simulink model "IndicatingResistor_Test"  (R2019a)
settings: Solver=VariableStepAuto  StartTime=0.0  StopTime=10.0  RelTol=1e-3
libraries: Murphy_SimscapeElectrical x6, fl_lib x1, nesl_utility x1, ee_lib x1
settings Model: Creator=Matt  LastModifiedBy=Matt
settings SimscapeCC: SimscapeLogType=all

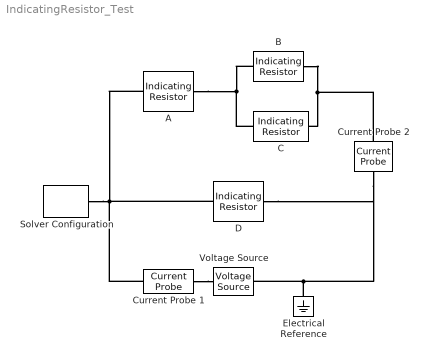
== system IndicatingResistor_Test ==
  A : Murphy_SimscapeElectrical/Indicating Resistor  amps=0.6  volts=6  resistance=10
      settings: SourceProductName=Simscape Electrical - Murphy Utilities
  B : Murphy_SimscapeElectrical/Indicating Resistor  amps=0.3  volts=3  resistance=10
      settings: SourceProductName=Simscape Electrical - Murphy Utilities
  C : Murphy_SimscapeElectrical/Indicating Resistor  amps=0.3  volts=3  resistance=10
      settings: SourceProductName=Simscape Electrical - Murphy Utilities
  Current Probe 1 : Murphy_SimscapeElectrical/Current Probe 
      settings: SourceProductName=Simscape Electrical - Murphy Utilities
  Current Probe 2 : Murphy_SimscapeElectrical/Current Probe 
      settings: SourceProductName=Simscape Electrical - Murphy Utilities
  D : Murphy_SimscapeElectrical/Indicating Resistor  amps=0.9  volts=9  resistance=10
      settings: SourceProductName=Simscape Electrical - Murphy Utilities
  Electrical Reference : fl_lib/Electrical/Electrical Elements/Electrical Reference
  Solver Configuration : nesl_utility/Solver Configuration  PhysicalDomain=network_engine_domain  SubClassName=solver  LeftPortType=input  RightPortType=generic  Tones=[]  Harmonics=[]  SimulateNoise=off  Profile=off  UseLocalSampling=off  EnableSwitchedLinearOptims=on  FrequencyDomain=off  UseCCode=off  RelTol=0.001  AbsTol=1e-06  MinStep=1e-09  ToWorkspace=off  RevertToSquareIcSolve=off  NumHomotopyIterations=100  PhasorMode=off  PhasorModeNumHarmonics=1  DoDC=on  ResidualTolerance=1e-09  UseLocalSolver=off  LocalSolverChoice=NE_BACKWARD_EULER_ADVANCER  LocalSolverSampleTime=0.001  DoFixedCost=off  MaxNonlinIter=3  MaxModeIter=2  LinearAlgebra=auto  EquationFormulation=NE_TIME_EF  DelaysMemoryBudget=1024  AutomaticFiltering=on  FilteringTimeConstant=0.001  PartitionStorageMethod=AS_NEEDED  PartitionMemoryBudget=1024  PartitionMethod=ROBUST
  Voltage Source : ee_lib/Sources/Voltage Source  dc_voltage=9 V  ac_voltage=0 V  ac_shift=0 rad  ac_frequency=60 Hz  noise_mode=0  PSD=0 V^2/Hz  repeatability=1  auto_seed=3394773151  user_seed=0  sample_time=1e-3 s  i_specify=off  i_priority=None  i=0 A  i_nominal_specify=off  i_nominal_unit=A  i_nominal_value=1  v_specify=off  v_priority=None  v=0 V  v_nominal_specify=off  v_nominal_unit=V  v_nominal_value=1
      settings: SourceProductName=Simscape Electrical
  connections:
  Electrical Reference/LConn1 -- D/RConn1 -- Current Probe 2/RConn1 -- Voltage Source/RConn1
  Current Probe 1/LConn1 -- Voltage Source/LConn1
  Current Probe 2/LConn1 -- C/RConn1 -- B/RConn1
  A/RConn1 -- C/LConn1 -- B/LConn1
  Solver Configuration/RConn1 -- D/LConn1 -- Current Probe 1/RConn1 -- A/LConn1
